simulink library "csc_vac_gimbal_steering_vernier_roll_acs_ctrl_lib"  (R2015b)
settings: Solver=ode45  StartTime=0.0  StopTime=10.0  RelTol=1e-3
values from neighbouring files (symbols this model uses):
  Kd = vac_gim_kd    [csc_vac_gimbal_vernier_roll_acs_ctrl_prep.m]
  Ki = vac_gim_ki    [csc_vac_gimbal_vernier_roll_acs_ctrl_prep.m]
  Kp = vac_gim_kp    [csc_vac_gimbal_vernier_roll_acs_ctrl_prep.m]
  vac_alpha_gain = 0.2    [csc_vac_vernier_acs_ctrl_init.m]
  vac_gim_x_act_c1 = 0.1    [csc_vac_gimbal_vernier_roll_acs_ctrl_init.m]
  vac_gim_x_act_c2 = 0.2    [csc_vac_gimbal_vernier_roll_acs_ctrl_init.m]
  vac_gim_x_act_lx1c = 0.3    [csc_vac_gimbal_vernier_roll_acs_ctrl_init.m]
  vac_gim_x_act_lz1c = 0.4    [csc_vac_gimbal_vernier_roll_acs_ctrl_init.m]
  vac_gim_y_act_c1 = 0.1    [csc_vac_gimbal_vernier_roll_acs_ctrl_init.m]
  vac_gim_y_act_c2 = 0.2    [csc_vac_gimbal_vernier_roll_acs_ctrl_init.m]
  vac_gim_y_act_ly1c = 0.3    [csc_vac_gimbal_vernier_roll_acs_ctrl_init.m]
  vac_gim_y_act_lz1c = 0.4    [csc_vac_gimbal_vernier_roll_acs_ctrl_init.m]
  vac_rotz_deadband = 1*pi/180    (= 0.0174532925199)    [csc_vac_vernier_acs_ctrl_init.m]
  vac_rotz_deadband_minus = 1*pi/180    (= 0.0174532925199)    [csc_vac_vernier_acs_ctrl_init.m]
  vac_thruster_alloc_vernier_x_minus = [16,24]    [csc_vac_vernier_acs_ctrl_init.m]
  vac_thruster_alloc_vernier_x_plus = [18,22]    [csc_vac_vernier_acs_ctrl_init.m]
  vac_thruster_alloc_vernier_y_minus = [15,19]    [csc_vac_vernier_acs_ctrl_init.m]
  vac_thruster_alloc_vernier_y_plus = [13,21]    [csc_vac_vernier_acs_ctrl_init.m]
  vac_thruster_alloc_vernier_z_minus = [14,20]    [csc_vac_vernier_acs_ctrl_init.m]
  vac_thruster_alloc_vernier_z_plus = [17,23]    [csc_vac_vernier_acs_ctrl_init.m]
undefined symbols (not defined in the file or in its folder): DiscIntNeverNeededParam, emp_inertia_wet_dry, emp_mass_wet_dry, vac_vernier_thruster_trq_z
libraries: util_info_lib x1, csu_ppd_phase_plane_distance_lib x1, csu_ptc_vernier_phaseplane_thruster_alloc_lib x1
settings Model: Creator=Nilesh  LastModifiedBy=jimkaidy
settings DataIOCC: SaveFormat=Array
settings DebuggingCC: UnderspecifiedInitializationDetection=Classic  MergeDetectMultiDrivingBlocksExec=none  SolverPrmCheckMsg=warning  StateNameClashWarn=warning
settings HardwareCC: ProdBitPerPointer=32  ProdLargestAtomicFloat=None  ProdIntDivRoundTo=Undefined  ProdEndianess=Unspecified  ProdWordSize=32  ProdHWDeviceType=32-bit Generic
settings GRTTargetCC: GeneratePreprocessorConditionals=Disable all
settings ConfigComp: CovModelRefEnable=Off  CovSFcnEnable=off

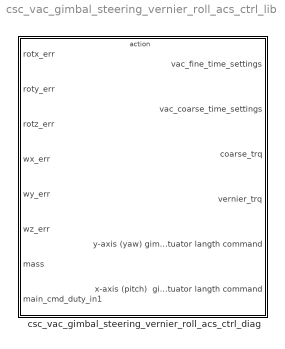
== system csc_vac_gimbal_steering_vernier_roll_acs_ctrl_lib ==
  csc_vac_gimbal_steering_vernier_roll_acs_ctrl_diag : Subsystem

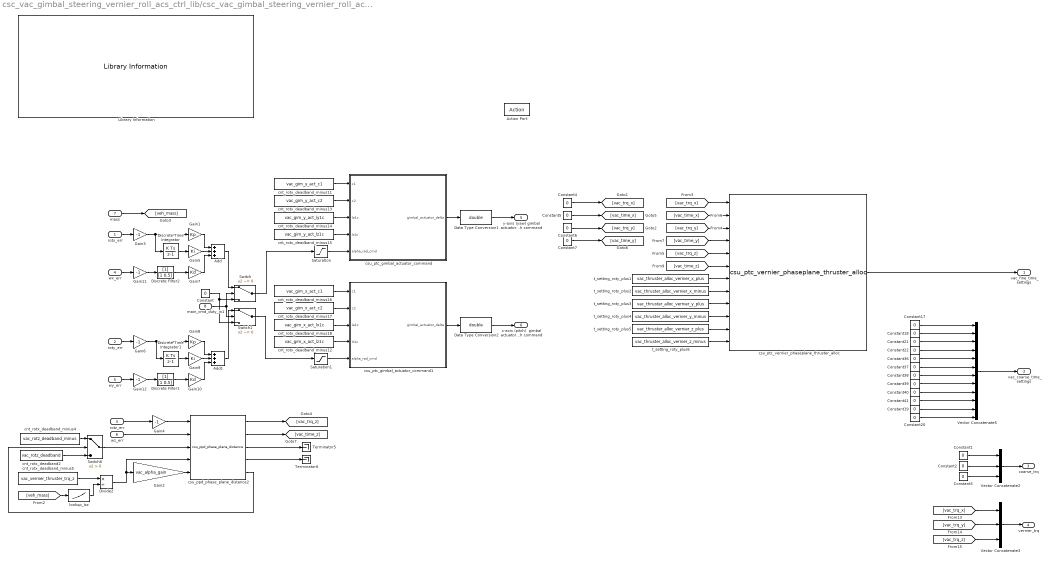
== system csc_vac_gimbal_steering_vernier_roll_acs_ctrl_lib/csc_vac_gimbal_steering_vernier_roll_acs_ctrl_diag ==
  rotx_err : Inport
  roty_err : Inport  Port=2
  rotz_err : Inport  Port=3
  wx_err : Inport  Port=4
  wy_err : Inport  Port=5
  wz_err : Inport  Port=6
  mass : Inport  Port=7
  main_cmd_duty_in1 : Inport  Port=8
  Action Port : ActionPort
  Add : Sum  Inputs=+++
  Add1 : Sum  Inputs=+++
  Constant : Constant  Value=0
  Constant{1..7} (7 alike) : Constant  Value=0  OutDataTypeStr=int8
  Constant{17..22,36..41} (12 alike) : Constant  Value=0  OutDataTypeStr=uint8
  Data Type Conversion1 : DataTypeConversion  OutDataTypeStr=double
  Data Type Conversion2 : DataTypeConversion  OutDataTypeStr=double
  Discrete Filter1 : DiscreteFilter
  Discrete Filter2 : DiscreteFilter
  Discrete-Time Integrator : DiscreteIntegrator  InitialConditionSetting=State (most efficient)  SampleTime=-1  ICPrevOutput=DiscIntNeverNeededParam  ICPrevScaledInput=DiscIntNeverNeededParam
  Discrete-Time Integrator1 : DiscreteIntegrator  InitialConditionSetting=State (most efficient)  SampleTime=-1  ICPrevOutput=DiscIntNeverNeededParam  ICPrevScaledInput=DiscIntNeverNeededParam
  Divide2 : Product  Inputs=*/
  Gain1 : Gain  Gain=Kp
  Gain10 : Gain  Gain=Kd
  Gain{3..4,6,11..12} (5 alike) : Gain  Gain=-1
  Gain2 : Gain  Gain=vac_alpha_gain
  Gain5 : Gain  Gain=Ki
  Gain7 : Gain  Gain=Kd
  Gain8 : Gain  Gain=Kp
  Gain9 : Gain  Gain=Ki
  Library Information : util_info_lib/Library Information  owner='NONE'
  Saturation : Saturate  UpperLimit=pi/2  LowerLimit=-pi/2
  Saturation1 : Saturate  UpperLimit=pi/2  LowerLimit=-pi/2
  Switch : Switch  Criteria=u2 ~= 0
  Switch1 : Switch  Criteria=u2 ~= 0
  Switch6 : Switch  Criteria=u2 > Threshold
  Terminator5 : Terminator
  Terminator6 : Terminator
  Vector Concatenate2 : Concatenate  NumInputs=3
  Vector Concatenate3 : Concatenate  NumInputs=3
  Vector Concatenate5 : Concatenate  NumInputs=12
  cnt_rotx_deadband2 : Constant  Value=vac_rotz_deadband
  cnt_rotx_deadband_minus11 : Constant  Value=vac_gim_y_act_c1
  cnt_rotx_deadband_minus12 : Constant  Value=vac_gim_x_act_lz1c
  cnt_rotx_deadband_minus13 : Constant  Value=vac_gim_y_act_c2
  cnt_rotx_deadband_minus14 : Constant  Value=vac_gim_y_act_ly1c
  cnt_rotx_deadband_minus15 : Constant  Value=vac_gim_y_act_lz1c
  cnt_rotx_deadband_minus16 : Constant  Value=vac_gim_x_act_c1
  cnt_rotx_deadband_minus17 : Constant  Value=vac_gim_x_act_c2
  cnt_rotx_deadband_minus18 : Constant  Value=vac_gim_x_act_lx1c
  cnt_rotx_deadband_minus4 : Constant  Value=vac_rotz_deadband_minus
  cnt_rotx_deadband_minus5 : Constant  Value=vac_vernier_thruster_trq_z
  csu_ppd_phase_plane_distance2 : csu_ppd_phase_plane_distance_lib/csu_ppd_phase_plane_distance
  csu_ptc_gimbal_actuator_command : MATLAB Function  TreatAsAtomicUnit=on
  csu_ptc_gimbal_actuator_command1 : MATLAB Function  TreatAsAtomicUnit=on
  csu_ptc_vernier_phaseplane_thruster_alloc : csu_ptc_vernier_phaseplane_thruster_alloc_lib/csu_ptc_vernier_phaseplane_thruster_alloc
  lookup_Izz : Lookup  InputValues=emp_mass_wet_dry  Table=emp_inertia_wet_dry(3,:)
  t_setting_roty_plus1 : Constant  Value=vac_thruster_alloc_vernier_x_plus
  t_setting_roty_plus2 : Constant  Value=vac_thruster_alloc_vernier_x_minus
  t_setting_roty_plus3 : Constant  Value=vac_thruster_alloc_vernier_y_plus
  t_setting_roty_plus4 : Constant  Value=vac_thruster_alloc_vernier_y_minus
  t_setting_roty_plus5 : Constant  Value=vac_thruster_alloc_vernier_z_plus
  t_setting_roty_plus6 : Constant  Value=vac_thruster_alloc_vernier_z_minus
  vac_fine_time_settings : Outport  OutputWhenDisabled=reset  InitialOutput=0
  vac_coarse_time_settings : Outport  Port=2  OutputWhenDisabled=reset  InitialOutput=0
  coarse_trq : Outport  Port=3  OutputWhenDisabled=reset  InitialOutput=0
  vernier_trq : Outport  Port=4  OutputWhenDisabled=reset  InitialOutput=0
  y-axis (yaw) gimbal actuator langth command : Outport  Port=5  OutputWhenDisabled=reset  InitialOutput=0
  x-axis (pitch)  gimbal actuator langth command : Outport  Port=6  OutputWhenDisabled=reset  InitialOutput=0
  wires:
  csu_ppd_phase_plane_distance2/3 -> Terminator5/1
  csu_ppd_phase_plane_distance2/4 -> Terminator6/1
  csu_ptc_vernier_phaseplane_thruster_alloc/1 -> vac_fine_time_settings/1
  [vac_time_y] -> csu_ptc_vernier_phaseplane_thruster_alloc/4
  [vac_time_z] -> csu_ptc_vernier_phaseplane_thruster_alloc/6
  [vac_time_x] -> csu_ptc_vernier_phaseplane_thruster_alloc/2
  t_setting_roty_plus6/1 -> csu_ptc_vernier_phaseplane_thruster_alloc/12
  t_setting_roty_plus5/1 -> csu_ptc_vernier_phaseplane_thruster_alloc/11
  t_setting_roty_plus4/1 -> csu_ptc_vernier_phaseplane_thruster_alloc/10
  t_setting_roty_plus3/1 -> csu_ptc_vernier_phaseplane_thruster_alloc/9
  t_setting_roty_plus2/1 -> csu_ptc_vernier_phaseplane_thruster_alloc/8
  t_setting_roty_plus1/1 -> csu_ptc_vernier_phaseplane_thruster_alloc/7
  [vac_trq_z] -> csu_ptc_vernier_phaseplane_thruster_alloc/5
  [vac_trq_y] -> csu_ptc_vernier_phaseplane_thruster_alloc/3
  [vac_trq_x] -> csu_ptc_vernier_phaseplane_thruster_alloc/1
  csu_ppd_phase_plane_distance2/2 -> [vac_time_z]
  Constant7/1 -> [vac_time_y]
  Constant5/1 -> [vac_time_x]
  Gain4/1 -> csu_ppd_phase_plane_distance2/1
  Gain3/1 -> Gain1/1, Discrete-Time Integrator/1
  csu_ppd_phase_plane_distance2/1 -> [vac_trq_z]
  Constant6/1 -> [vac_trq_y]
  Constant4/1 -> [vac_trq_x]
  Gain2/1 -> csu_ppd_phase_plane_distance2/5
  Divide2/1 -> csu_ppd_phase_plane_distance2/4, Gain2/1
  cnt_rotx_deadband_minus5/1 -> Divide2/1
  lookup_Izz/1 -> Divide2/2
  [veh_mass] -> lookup_Izz/1
  csu_ppd_phase_plane_distance2/5 -> Switch6/2
  cnt_rotx_deadband_minus4/1 -> Switch6/1
  cnt_rotx_deadband2/1 -> Switch6/3
  Switch6/1 -> csu_ppd_phase_plane_distance2/3
  mass/1 -> [veh_mass]
  wz_err/1 -> csu_ppd_phase_plane_distance2/2
  rotz_err/1 -> Gain4/1
  roty_err/1 -> Gain6/1
  wx_err/1 -> Gain11/1
  Constant3/1 -> Vector Concatenate2/3
  Vector Concatenate2/1 -> coarse_trq/1
  Constant2/1 -> Vector Concatenate2/2
  Constant1/1 -> Vector Concatenate2/1
  [vac_trq_z] -> Vector Concatenate3/3
  Vector Concatenate3/1 -> vernier_trq/1
  [vac_trq_y] -> Vector Concatenate3/2
  [vac_trq_x] -> Vector Concatenate3/1
  Constant17/1 -> Vector Concatenate5/1
  Constant20/1 -> Vector Concatenate5/12
  Constant18/1 -> Vector Concatenate5/2
  Constant19/1 -> Vector Concatenate5/11
  Constant21/1 -> Vector Concatenate5/3
  Constant22/1 -> Vector Concatenate5/4
  Constant41/1 -> Vector Concatenate5/10
  Constant40/1 -> Vector Concatenate5/9
  Constant36/1 -> Vector Concatenate5/5
  Constant37/1 -> Vector Concatenate5/6
  Constant39/1 -> Vector Concatenate5/8
  Constant38/1 -> Vector Concatenate5/7
  Vector Concatenate5/1 -> vac_coarse_time_settings/1
  Discrete-Time Integrator/1 -> Gain5/1
  Gain1/1 -> Add/1
  Gain5/1 -> Add/2
  Gain6/1 -> Discrete-Time Integrator1/1, Gain8/1
  wy_err/1 -> Gain12/1
  Discrete-Time Integrator1/1 -> Gain9/1
  Gain8/1 -> Add1/1
  Gain9/1 -> Add1/2
  cnt_rotx_deadband_minus11/1 -> csu_ptc_gimbal_actuator_command/1(c1)
  cnt_rotx_deadband_minus13/1 -> csu_ptc_gimbal_actuator_command/2(c2)
  cnt_rotx_deadband_minus14/1 -> csu_ptc_gimbal_actuator_command/3(la1c)
  cnt_rotx_deadband_minus15/1 -> csu_ptc_gimbal_actuator_command/4(lz1c)
  csu_ptc_gimbal_actuator_command/1(gimbal_actuator_delta) -> Data Type Conversion1/1
  cnt_rotx_deadband_minus16/1 -> csu_ptc_gimbal_actuator_command1/1(c1)
  cnt_rotx_deadband_minus17/1 -> csu_ptc_gimbal_actuator_command1/2(c2)
  cnt_rotx_deadband_minus18/1 -> csu_ptc_gimbal_actuator_command1/3(la1c)
  cnt_rotx_deadband_minus12/1 -> csu_ptc_gimbal_actuator_command1/4(lz1c)
  Switch/1 -> Saturation/1
  csu_ptc_gimbal_actuator_command1/1(gimbal_actuator_delta) -> Data Type Conversion2/1
  Saturation/1 -> csu_ptc_gimbal_actuator_command/5(alpha_rad_cmd)
  Saturation1/1 -> csu_ptc_gimbal_actuator_command1/5(alpha_rad_cmd)
  rotx_err/1 -> Gain3/1
  Gain7/1 -> Add/3
  Gain10/1 -> Add1/3
  Gain11/1 -> Discrete Filter2/1
  Discrete Filter2/1 -> Gain7/1
  Gain12/1 -> Discrete Filter1/1
  Discrete Filter1/1 -> Gain10/1
  main_cmd_duty_in1/1 -> Switch/2, Switch1/2
  Switch1/1 -> Saturation1/1
  Constant/1 -> Switch1/3, Switch/3
  Add/1 -> Switch/1
  Add1/1 -> Switch1/1
  Data Type Conversion1/1 -> y-axis (yaw) gimbal actuator langth command/1
  Data Type Conversion2/1 -> x-axis (pitch)  gimbal actuator langth command/1

== matlab function csc_vac_gimbal_steering_vernier_roll_acs_ctrl_lib/csc_vac_gimbal_steering_vernier_roll_acs_ctrl_diag/csu_ptc_gimbal_actuator_command1 ==
  data: c1 input; gimbal_actuator_delta output; c2 input; la1c input; lz1c input; alpha_rad_cmd input
function gimbal_actuator_delta = gimbal_command(c1,c2,la1c,lz1c,alpha_rad_cmd)
%#codegen

Rmount = sqrt(c1^2 + c2^2);

Lcmd = sqrt((la1c - Rmount*sqrt(1 - 1/(1+(tan(alpha_rad_cmd) + c1/c2)^2)))^2 + (lz1c + Rmount/sqrt(1+(tan(alpha_rad_cmd)+c1/c2)^2))^2);

Lo = sqrt((la1c - c1)^2 + (lz1c + c2)^2);

Lerr =( Lcmd - Lo);

gimbal_actuator_delta = Lerr;

== matlab function csc_vac_gimbal_steering_vernier_roll_acs_ctrl_lib/csc_vac_gimbal_steering_vernier_roll_acs_ctrl_diag/csu_ptc_gimbal_actuator_command ==
  data: c1 input; gimbal_actuator_delta output; c2 input; la1c input; lz1c input; alpha_rad_cmd input
function gimbal_actuator_delta = gimbal_command(c1,c2,la1c,lz1c,alpha_rad_cmd)
%#codegen

Rmount = sqrt(c1^2 + c2^2);

Lcmd = sqrt((la1c - Rmount*sqrt(1 - 1/(1+(tan(alpha_rad_cmd) + c1/c2)^2)))^2 + (lz1c + Rmount/sqrt(1+(tan(alpha_rad_cmd)+c1/c2)^2))^2);

Lo = sqrt((la1c - c1)^2 + (lz1c + c2)^2);

Lerr =( Lcmd - Lo);

gimbal_actuator_delta = Lerr;
